simulink model "Lab04Exp"  (Simulink 7.1)
settings: Solver=ode45  StartTime=0.0  StopTime=10.0  RelTol=1e-3
settings Model: Creator=George  LastModifiedBy=George

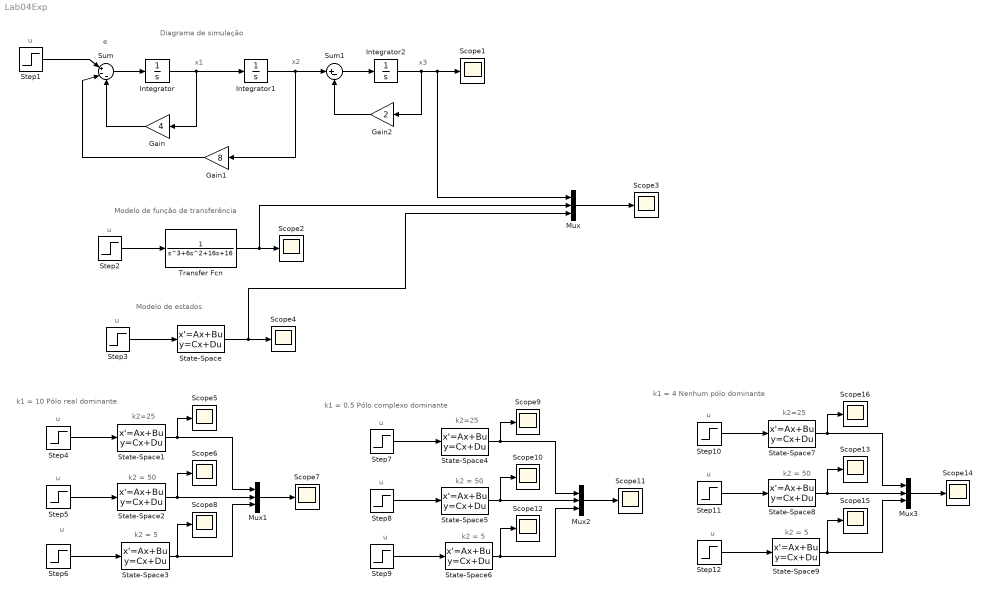
== system Lab04Exp ==
  note: x1
  note: x2
  note: x3
  note: u
  note: e
  note: u
  note: u
  note: u
  note: u
  note: u
  note: u
  note: u
  note: u
  note: k1 = 10
      | Pólo real dominante
  note: u
  note: u
  note: u
  note: k1 = 0.5
      | Pólo complexo dominante
  note: k1 = 4
      | Nenhum pólo dominante
  note: k2=25
  note: k2 = 50
  note: k2 = 5
  note: k2=25
  note: k2=25
  note: k2 = 50
  note: k2 = 50
  note: k2 = 5
  note: k2 = 5
  note: Diagrama de simulação
  note: Modelo de função de transferência
  note: Modelo de estados
  Gain : Gain  Orientation=left  Gain=4  ParameterDataType=sfix(16)  ParameterScaling=2^0  OutDataType=sfix(16)  OutScaling=2^0
  Gain1 : Gain  Orientation=left  Gain=8  ParameterDataType=sfix(16)  ParameterScaling=2^0  OutDataType=sfix(16)  OutScaling=2^0
  Gain2 : Gain  Orientation=left  Gain=2  ParameterDataType=sfix(16)  ParameterScaling=2^0  OutDataType=sfix(16)  OutScaling=2^0
  Integrator : Integrator
  Integrator1 : Integrator
  Integrator2 : Integrator
  Mux{,1..3} (4 alike) : Mux  Inputs=3
  Scope{1..16} (16 alike) : Scope
      Scope10 settings: SaveName=ScopeData8
      Scope11 settings: SaveName=ScopeData9
      Scope12 settings: SaveName=ScopeData10
      Scope13 settings: SaveName=ScopeData12
      Scope14 settings: SaveName=ScopeData13
      Scope15 settings: SaveName=ScopeData14
      Scope16 settings: SaveName=ScopeData15
      Scope3 settings: SaveName=ScopeData2
      Scope4 settings: SaveName=ScopeData3
      Scope5 settings: SaveName=ScopeData4
      Scope6 settings: SaveName=ScopeData5
      Scope7 settings: SaveName=ScopeData6
      Scope8 settings: SaveName=ScopeData7
      Scope9 settings: SaveName=ScopeData11
  State-Space : StateSpace  A=[-4 -8 0; 1 0 0; 0 1 -2]  B=[1; 0; 0]  C=[0 0 1]  D=0
  State-Space1 : StateSpace  A=[-10 -25 0; 1 0 0; 0 1 -2]  B=[1; 0; 0]  C=[0 0 50]  D=0
  State-Space2 : StateSpace  A=[-10 -50 0; 1 0 0; 0 1 -2]  B=[1; 0; 0]  C=[0 0 50]  D=0
  State-Space3 : StateSpace  A=[-10 -5 0; 1 0 0; 0 1 -2]  B=[1; 0; 0]  C=[0 0 50]  D=0
  State-Space4 : StateSpace  A=[-0.5 -25 0; 1 0 0; 0 1 -2]  B=[1; 0; 0]  C=[0 0 50]  D=0
  State-Space5 : StateSpace  A=[-0.5 -50 0; 1 0 0; 0 1 -2]  B=[1; 0; 0]  C=[0 0 50]  D=0
  State-Space6 : StateSpace  A=[-0.5 -5 0; 1 0 0; 0 1 -2]  B=[1; 0; 0]  C=[0 0 50]  D=0
  State-Space7 : StateSpace  A=[-4 -25 0; 1 0 0; 0 1 -2]  B=[1; 0; 0]  C=[0 0 50]  D=0
  State-Space8 : StateSpace  A=[-4 -50 0; 1 0 0; 0 1 -2]  B=[1; 0; 0]  C=[0 0 50]  D=0
  State-Space9 : StateSpace  A=[-4 -5 0; 1 0 0; 0 1 -2]  B=[1; 0; 0]  C=[0 0 50]  D=0
  Step{1..12} (12 alike) : Step  Time=0  SampleTime=0
  Sum : Sum  Inputs=|+--  OutDataType=sfix(16)  OutScaling=2^0
  Sum1 : Sum  Inputs=|+-  OutDataType=sfix(16)  OutScaling=2^0
  Transfer Fcn : TransferFcn  Denominator=[1 6 16 16]
  wires:
  Step1/1 -> Sum/1
  Sum/1 -> Integrator/1
  Integrator/1 -> Integrator1/1, Gain/1
  Integrator1/1 -> Sum1/1, Gain1/1
  Sum1/1 -> Integrator2/1
  Integrator2/1 -> Gain2/1, Scope1/1, Mux/1
  Gain/1 -> Sum/3
  Gain1/1 -> Sum/2
  Gain2/1 -> Sum1/2
  Step2/1 -> Transfer Fcn/1
  Transfer Fcn/1 -> Scope2/1, Mux/2
  Step3/1 -> State-Space/1
  State-Space/1 -> Scope4/1, Mux/3
  Mux/1 -> Scope3/1
  Step4/1 -> State-Space1/1
  Step5/1 -> State-Space2/1
  Step6/1 -> State-Space3/1
  State-Space1/1 -> Mux1/1, Scope5/1
  State-Space2/1 -> Mux1/2, Scope6/1
  State-Space3/1 -> Mux1/3, Scope8/1
  Mux1/1 -> Scope7/1
  Step7/1 -> State-Space4/1
  Step8/1 -> State-Space5/1
  Step9/1 -> State-Space6/1
  State-Space4/1 -> Mux2/1, Scope9/1
  State-Space5/1 -> Mux2/2, Scope10/1
  State-Space6/1 -> Mux2/3, Scope12/1
  Mux2/1 -> Scope11/1
  Step10/1 -> State-Space7/1
  Step11/1 -> State-Space8/1
  Step12/1 -> State-Space9/1
  State-Space7/1 -> Mux3/1, Scope16/1
  State-Space8/1 -> Mux3/2, Scope13/1
  State-Space9/1 -> Mux3/3, Scope15/1
  Mux3/1 -> Scope14/1
